simulink model "PID_controller"  (R2020b)
settings: Solver=ode15s  StartTime=0.0  StopTime=0.2  RelTol=1e-3
settings Model: Creator=priyaD  LastModifiedBy=priyaD
settings DataIOCC: SaveOutput=off  SaveTime=off

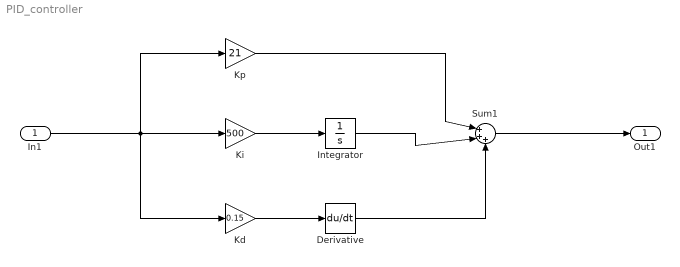
== system PID_controller ==
  In1 : Inport  OutDataTypeStr=double  PortDimensions=1  SampleTime=0
  Derivative : Derivative
  Integrator : Integrator
  Kd : Gain  Gain=0.15
  Ki : Gain  Gain=500
  Kp : Gain  Gain=21
  Sum1 : Sum  Inputs=|+++
  Out1 : Outport  OutDataTypeStr=double  PortDimensions=1  SampleTime=0
  wires:
  In1/1 -> Kp/1, Ki/1, Kd/1
  Integrator/1 -> Sum1/2
  Sum1/1 -> Out1/1
  Derivative/1 -> Sum1/3
  Ki/1 -> Integrator/1
  Kp/1 -> Sum1/1
  Kd/1 -> Derivative/1
